simulink model "EFR_Probe"  (R2021a)
settings: Solver=VariableStepAuto  StartTime=0.0  StopTime=8  RelTol=1e-3
undefined symbols (not defined in the file or in its folder): f_serv_low, f_serv_upp, P_serv_low, P_serv_upp
libraries: simulink x3
settings Model: Creator=Sergio Cantillo  LastModifiedBy=Sergio Cantillo

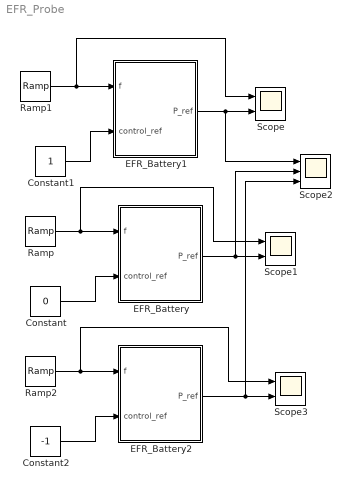
== system EFR_Probe ==
  Constant : Constant  Value=0
  Constant1 : Constant
  Constant2 : Constant  Value=-1
  EFR_Battery : Subsystem
  EFR_Battery1 : Subsystem
  EFR_Battery2 : Subsystem
  Ramp : simulink/Sources/Ramp  slope=0.25  start=0  InitialOutput=49
  Ramp1 : simulink/Sources/Ramp  slope=0.25  start=0  InitialOutput=49
  Ramp2 : simulink/Sources/Ramp  slope=0.25  start=0  InitialOutput=49
  Scope : Scope  NumInputPorts=2
  Scope1 : Scope  NumInputPorts=2
  Scope2 : Scope  NumInputPorts=3
  Scope3 : Scope  NumInputPorts=2
  wires:
  Ramp/1 -> Scope1/1, EFR_Battery/1(f)
  Constant/1 -> EFR_Battery/2(control_ref)
  Ramp1/1 -> Scope/1, EFR_Battery1/1(f)
  Constant1/1 -> EFR_Battery1/2(control_ref)
  EFR_Battery1/1(P_ref) -> Scope2/1, Scope/2
  EFR_Battery/1(P_ref) -> Scope2/2, Scope1/2
  EFR_Battery2/1(P_ref) -> Scope3/2, Scope2/3
  Constant2/1 -> EFR_Battery2/2(control_ref)
  Ramp2/1 -> Scope3/1, EFR_Battery2/1(f)

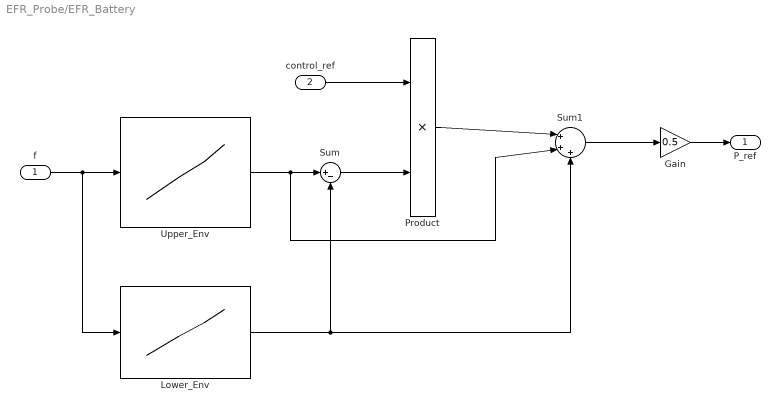
== system EFR_Probe/EFR_Battery ==
  f : Inport
  control_ref : Inport  Port=2  SampleTime=10
  Gain : Gain  Gain=0.5
  Lower_Env : Lookup_n-D  NumberOfTableDimensions=1  BreakpointsForDimension1=f_serv_low  Table=P_serv_low  ExtrapMethod=Clip  UseLastTableValue=on  InternalRulePriority=Speed  RndMeth=Simplest  InputSameDT=on
  Product : Product
  Sum : Sum  Inputs=|+-
  Sum1 : Sum  Inputs=|+++
  Upper_Env : Lookup_n-D  NumberOfTableDimensions=1  BreakpointsForDimension1=f_serv_upp  Table=P_serv_upp  ExtrapMethod=Clip  UseLastTableValue=on  InternalRulePriority=Speed  RndMeth=Simplest  InputSameDT=on
  P_ref : Outport  VectorParamsAs1DForOutWhenUnconnected=off
  wires:
  f/1 -> Lower_Env/1, Upper_Env/1
  control_ref/1 -> Product/1
  Lower_Env/1 -> Sum1/3, Sum/2
  Gain/1 -> P_ref/1
  Sum/1 -> Product/2
  Product/1 -> Sum1/1
  Sum1/1 -> Gain/1
  Upper_Env/1 -> Sum/1, Sum1/2

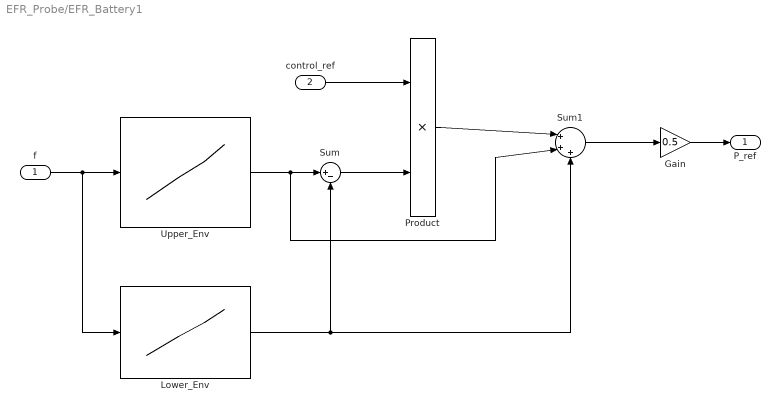
== system EFR_Probe/EFR_Battery1 ==
  f : Inport
  control_ref : Inport  Port=2  SampleTime=10
  Gain : Gain  Gain=0.5
  Lower_Env : Lookup_n-D  NumberOfTableDimensions=1  BreakpointsForDimension1=f_serv_low  Table=P_serv_low  ExtrapMethod=Clip  UseLastTableValue=on  InternalRulePriority=Speed  RndMeth=Simplest  InputSameDT=on
  Product : Product
  Sum : Sum  Inputs=|+-
  Sum1 : Sum  Inputs=|+++
  Upper_Env : Lookup_n-D  NumberOfTableDimensions=1  BreakpointsForDimension1=f_serv_upp  Table=P_serv_upp  ExtrapMethod=Clip  UseLastTableValue=on  InternalRulePriority=Speed  RndMeth=Simplest  InputSameDT=on
  P_ref : Outport  VectorParamsAs1DForOutWhenUnconnected=off
  wires:
  f/1 -> Lower_Env/1, Upper_Env/1
  control_ref/1 -> Product/1
  Lower_Env/1 -> Sum1/3, Sum/2
  Gain/1 -> P_ref/1
  Sum/1 -> Product/2
  Product/1 -> Sum1/1
  Sum1/1 -> Gain/1
  Upper_Env/1 -> Sum/1, Sum1/2

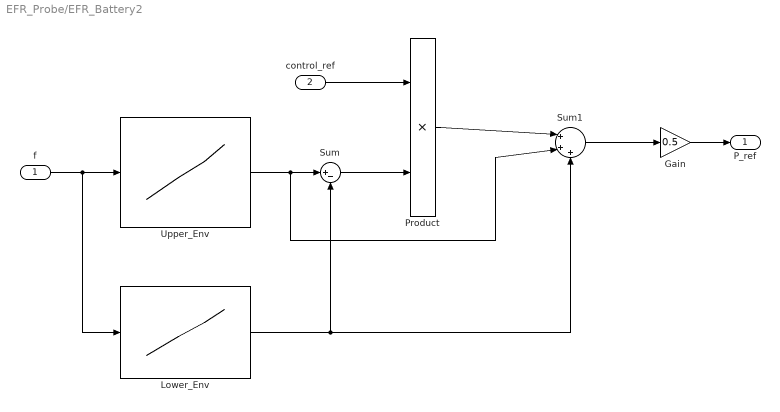
== system EFR_Probe/EFR_Battery2 ==
  f : Inport
  control_ref : Inport  Port=2  SampleTime=10
  Gain : Gain  Gain=0.5
  Lower_Env : Lookup_n-D  NumberOfTableDimensions=1  BreakpointsForDimension1=f_serv_low  Table=P_serv_low  ExtrapMethod=Clip  UseLastTableValue=on  InternalRulePriority=Speed  RndMeth=Simplest  InputSameDT=on
  Product : Product
  Sum : Sum  Inputs=|+-
  Sum1 : Sum  Inputs=|+++
  Upper_Env : Lookup_n-D  NumberOfTableDimensions=1  BreakpointsForDimension1=f_serv_upp  Table=P_serv_upp  ExtrapMethod=Clip  UseLastTableValue=on  InternalRulePriority=Speed  RndMeth=Simplest  InputSameDT=on
  P_ref : Outport  VectorParamsAs1DForOutWhenUnconnected=off
  wires:
  f/1 -> Lower_Env/1, Upper_Env/1
  control_ref/1 -> Product/1
  Lower_Env/1 -> Sum1/3, Sum/2
  Gain/1 -> P_ref/1
  Sum/1 -> Product/2
  Product/1 -> Sum1/1
  Sum1/1 -> Gain/1
  Upper_Env/1 -> Sum/1, Sum1/2
